simulink model "volo_agcdc_pipelined"  (R2012b)
settings: Solver=ode45  StartTime=0.0  StopTime=1000  RelTol=1e-3
PreLoadFcn:
  | volo_agcdc_init
InitFcn:
  | volo_agcdc_init
StartFcn:
  | volo_agcdc_init
values from neighbouring files (symbols this model uses):
  agc_idleState = 0    [volo_agcdc_init.m]
  agc_numAddrBits = agc_numOutputs + agc_numStateBits    [volo_agcdc_init.m]
  regDCRemoval_AvgLength = 64    [volo_agcdc_init.m]
  regSatDet_NumSamples = 16    [volo_agcdc_init.m]
undefined symbols (not defined in the file or in its folder): gcbh, xlBlockLoadCallback, xlGetNormalizedPeriod
libraries: xbsIndex_r4 x681, xbsEDKLib_r4 x1
(part 2 of 7)

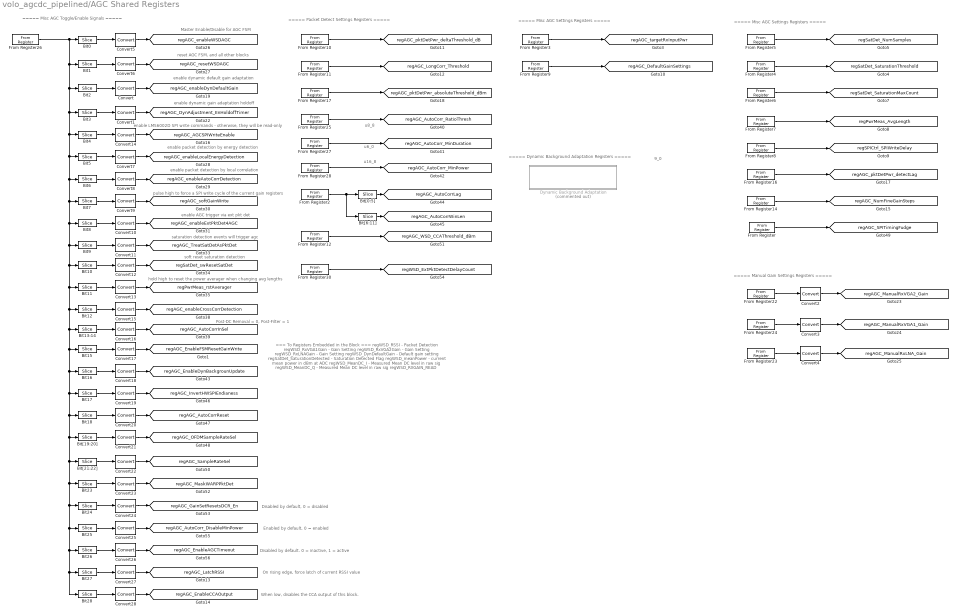
== system volo_agcdc_pipelined/AGC Shared Registers ==
  note: When low, disables the CCA output of this block.
  note: On rising edge, force latch of current RSSI value
  note: Disabled by default, 0 = disabled
  note: Enabled by default, 0 = enabled
  note: Disabled by default. 0 = inactive, 1 = active
  note: u6_0
  note: u16_8
  note: u8_8
  note: 9_0
  note: Post-DC Removal = 0, Post-Filter = 1
  note: ===== Misc AGC Toggle/Enable Signals =====
  note: ===== Dynamic Background Adaptation Registers =====
  note: ===== Misc AGC Settings Registers =====
  note: ===== Misc AGC Settings Registers =====
  note: ===== Packet Detect Settings Registers =====
  note: ===== Manual Gain Settings Registers =====
  note: saturation detection events will trigger agc
  note: enable AGC trigger via ext pkt det
  note: pulse high to force a SPI write cycle of the current gain registers
  note: enable packet detection by local correlation
  note: enable packet detection by energy detection
  note: enable LMS6002D SPI write commands - otherwise, they will be read-only
  note: enable dynamic gain adaptation holdoff
  note: enable dynamic default gain adaptation
  note: reset AGC FSM, and all other blocks
  note: Master Enable/Disable for AGC FSM
  note: === To Registers Embedded in the Block ===
      |
      | regWSD_RSSI - Packet Detection
      | regWSD_RxVGA1Gain - Gain Setting
      | regWSD_RxVGA2Gain - Gain Setting
      | regWSD_RxLNAGain - Gain Setting
      | regWSD_DynDefaultGain - Default gain setting
      | regSatDet_SaturationDetected - Saturation Detected Flag
      | regWSD_meanPower - current mean power in dBm at ADC
      | regWSD_MeanDC_I - Measured Mean DC level in raw sig
      | regWSD_MeanDC_Q - Measured Mean DC level in raw sig
      | regWSD_RXGAIN_READ
  note: soft reset saturation detection
  note: hold high to reset the power averager when changing avg lengths
  Bit0 : xbsIndex_r4/Slice  nbits=1  boolean_output=off  mode=Lower Bit Location + Width  bit1=0  base1=MSB of Input  bit0=0  base0=LSB of Input  dbl_ovrd=off  block_type=slice
  Bit1 : xbsIndex_r4/Slice  nbits=1  boolean_output=off  mode=Lower Bit Location + Width  bit1=0  base1=MSB of Input  bit0=1  base0=LSB of Input  dbl_ovrd=off  block_type=slice
  Bit10 : xbsIndex_r4/Slice  nbits=1  boolean_output=off  mode=Lower Bit Location + Width  bit1=0  base1=MSB of Input  bit0=10  base0=LSB of Input  dbl_ovrd=off  block_type=slice
  Bit11 : xbsIndex_r4/Slice  nbits=1  boolean_output=off  mode=Lower Bit Location + Width  bit1=0  base1=MSB of Input  bit0=11  base0=LSB of Input  dbl_ovrd=off  block_type=slice
  Bit12 : xbsIndex_r4/Slice  nbits=1  boolean_output=off  mode=Lower Bit Location + Width  bit1=0  base1=MSB of Input  bit0=12  base0=LSB of Input  dbl_ovrd=off  block_type=slice
  Bit13:14 : xbsIndex_r4/Slice  nbits=2  boolean_output=off  mode=Lower Bit Location + Width  bit1=0  base1=MSB of Input  bit0=13  base0=LSB of Input  dbl_ovrd=off  block_type=slice
  Bit15 : xbsIndex_r4/Slice  nbits=1  boolean_output=off  mode=Lower Bit Location + Width  bit1=0  base1=MSB of Input  bit0=15  base0=LSB of Input  dbl_ovrd=off  block_type=slice
  Bit16 : xbsIndex_r4/Slice  nbits=1  boolean_output=off  mode=Lower Bit Location + Width  bit1=0  base1=MSB of Input  bit0=16  base0=LSB of Input  dbl_ovrd=off  block_type=slice
  Bit17 : xbsIndex_r4/Slice  nbits=1  boolean_output=off  mode=Lower Bit Location + Width  bit1=0  base1=MSB of Input  bit0=17  base0=LSB of Input  dbl_ovrd=off  block_type=slice
  Bit18 : xbsIndex_r4/Slice  nbits=1  boolean_output=off  mode=Lower Bit Location + Width  bit1=0  base1=MSB of Input  bit0=18  base0=LSB of Input  dbl_ovrd=off  block_type=slice
  Bit2 : xbsIndex_r4/Slice  nbits=1  boolean_output=off  mode=Lower Bit Location + Width  bit1=0  base1=MSB of Input  bit0=2  base0=LSB of Input  dbl_ovrd=off  block_type=slice
  Bit23 : xbsIndex_r4/Slice  nbits=1  boolean_output=off  mode=Lower Bit Location + Width  bit1=0  base1=MSB of Input  bit0=23  base0=LSB of Input  dbl_ovrd=off  block_type=slice
  Bit24 : xbsIndex_r4/Slice  nbits=1  boolean_output=off  mode=Lower Bit Location + Width  bit1=0  base1=MSB of Input  bit0=24  base0=LSB of Input  dbl_ovrd=off  block_type=slice
  Bit25 : xbsIndex_r4/Slice  nbits=1  boolean_output=off  mode=Lower Bit Location + Width  bit1=0  base1=MSB of Input  bit0=25  base0=LSB of Input  dbl_ovrd=off  block_type=slice
  Bit26 : xbsIndex_r4/Slice  nbits=1  boolean_output=off  mode=Lower Bit Location + Width  bit1=0  base1=MSB of Input  bit0=26  base0=LSB of Input  dbl_ovrd=off  block_type=slice
  Bit27 : xbsIndex_r4/Slice  nbits=1  boolean_output=off  mode=Lower Bit Location + Width  bit1=0  base1=MSB of Input  bit0=27  base0=LSB of Input  dbl_ovrd=off  block_type=slice
  Bit28 : xbsIndex_r4/Slice  nbits=1  boolean_output=off  mode=Lower Bit Location + Width  bit1=0  base1=MSB of Input  bit0=28  base0=LSB of Input  dbl_ovrd=off  block_type=slice
  Bit3 : xbsIndex_r4/Slice  nbits=1  boolean_output=off  mode=Lower Bit Location + Width  bit1=0  base1=MSB of Input  bit0=3  base0=LSB of Input  dbl_ovrd=off  block_type=slice
  Bit4 : xbsIndex_r4/Slice  nbits=1  boolean_output=off  mode=Lower Bit Location + Width  bit1=0  base1=MSB of Input  bit0=4  base0=LSB of Input  dbl_ovrd=off  block_type=slice
  Bit5 : xbsIndex_r4/Slice  nbits=1  boolean_output=off  mode=Lower Bit Location + Width  bit1=0  base1=MSB of Input  bit0=5  base0=LSB of Input  dbl_ovrd=off  block_type=slice
  Bit6 : xbsIndex_r4/Slice  nbits=1  boolean_output=off  mode=Lower Bit Location + Width  bit1=0  base1=MSB of Input  bit0=6  base0=LSB of Input  dbl_ovrd=off  block_type=slice
  Bit7 : xbsIndex_r4/Slice  nbits=1  boolean_output=off  mode=Lower Bit Location + Width  bit1=0  base1=MSB of Input  bit0=7  base0=LSB of Input  dbl_ovrd=off  block_type=slice
  Bit8 : xbsIndex_r4/Slice  nbits=1  boolean_output=off  mode=Lower Bit Location + Width  bit1=0  base1=MSB of Input  bit0=8  base0=LSB of Input  dbl_ovrd=off  block_type=slice
  Bit9 : xbsIndex_r4/Slice  nbits=1  boolean_output=off  mode=Lower Bit Location + Width  bit1=0  base1=MSB of Input  bit0=9  base0=LSB of Input  dbl_ovrd=off  block_type=slice
  Bit[0:5] : xbsIndex_r4/Slice  nbits=6  boolean_output=off  mode=Lower Bit Location + Width  bit1=0  base1=MSB of Input  bit0=0  base0=LSB of Input  dbl_ovrd=off  block_type=slice
  Bit[19:20] : xbsIndex_r4/Slice  nbits=2  boolean_output=off  mode=Lower Bit Location + Width  bit1=0  base1=MSB of Input  bit0=19  base0=LSB of Input  dbl_ovrd=off  block_type=slice
  Bit[21:22] : xbsIndex_r4/Slice  nbits=2  boolean_output=off  mode=Lower Bit Location + Width  bit1=0  base1=MSB of Input  bit0=21  base0=LSB of Input  dbl_ovrd=off  block_type=slice
  Bit[6:11] : xbsIndex_r4/Slice  nbits=6  boolean_output=off  mode=Lower Bit Location + Width  bit1=0  base1=MSB of Input  bit0=6  base0=LSB of Input  dbl_ovrd=off  block_type=slice
  Convert{,1,5..15} (13 alike) : xbsIndex_r4/Convert  gui_display_data_type=Boolean  arith_type=Boolean  n_bits=16  bin_pt=14  float_type=Single  exp_bits=8  fraction_bits=24  quantization=Truncate  overflow=Wrap  en=off  latency=0  dbl_ovrd=off  pipeline=off  block_type=convert
  Convert16 : xbsIndex_r4/Convert  gui_display_data_type=Fixed-point  arith_type=Unsigned  n_bits=1  bin_pt=0  float_type=Single  exp_bits=8  fraction_bits=24  quantization=Truncate  overflow=Wrap  en=off  latency=0  dbl_ovrd=off  pipeline=off  block_type=convert
  Convert{17..20,23..28} (10 alike) : xbsIndex_r4/Convert  gui_display_data_type=Boolean  arith_type=Boolean  n_bits=2  bin_pt=0  float_type=Single  exp_bits=8  fraction_bits=24  quantization=Truncate  overflow=Wrap  en=off  latency=0  dbl_ovrd=off  pipeline=off  block_type=convert
  Convert2 : xbsIndex_r4/Convert  gui_display_data_type=Fixed-point  arith_type=Unsigned  n_bits=8  bin_pt=0  float_type=Single  exp_bits=8  fraction_bits=24  quantization=Truncate  overflow=Wrap  en=off  latency=0  dbl_ovrd=off  pipeline=off  block_type=convert
  Convert21 : xbsIndex_r4/Convert  gui_display_data_type=Fixed-point  arith_type=Unsigned  n_bits=2  bin_pt=0  float_type=Single  exp_bits=8  fraction_bits=24  quantization=Truncate  overflow=Wrap  en=off  latency=0  dbl_ovrd=off  pipeline=off  block_type=convert
  Convert22 : xbsIndex_r4/Convert  gui_display_data_type=Fixed-point  arith_type=Unsigned  n_bits=2  bin_pt=0  float_type=Single  exp_bits=8  fraction_bits=24  quantization=Truncate  overflow=Wrap  en=off  latency=0  dbl_ovrd=off  pipeline=off  block_type=convert
  Convert3 : xbsIndex_r4/Convert  gui_display_data_type=Fixed-point  arith_type=Unsigned  n_bits=8  bin_pt=0  float_type=Single  exp_bits=8  fraction_bits=24  quantization=Truncate  overflow=Wrap  en=off  latency=0  dbl_ovrd=off  pipeline=off  block_type=convert
  Convert4 : xbsIndex_r4/Convert  gui_display_data_type=Fixed-point  arith_type=Unsigned  n_bits=8  bin_pt=0  float_type=Single  exp_bits=8  fraction_bits=24  quantization=Truncate  overflow=Wrap  en=off  latency=0  dbl_ovrd=off  pipeline=off  block_type=convert
  Dynamic Background Adaptation : Subsystem  Commented=on
  From Register : xbsIndex_r4/From Register  shared_memory_name='regAGC_SPITIMINGFUDGE'  init=68  period=1  ownership=Locally owned and initialized  gui_display_data_type=Fixed-point  arith_type=Unsigned  n_bits=12  bin_pt=0  preci_type=Single  dbl_ovrd=off  block_type=fromreg
      settings: AttributesFormatString=<< %<shared_memory_name> >>  infoedit="Register block that reads data to a shared memory register.  Delay of one sample period."
  From Register10 : xbsIndex_r4/From Register  shared_memory_name='regAGC_pktDetPwr_deltaThreshold_dBm'  init=regAGC_pktDetPwr_deltaThreshold_dBm  period=1  ownership=Locally owned and initialized  gui_display_data_type=Fixed-point  arith_type="Signed  (2's comp)"  n_bits=9  bin_pt=0  preci_type=Single  dbl_ovrd=off  block_type=fromreg
      settings: AttributesFormatString=<< %<shared_memory_name> >>  infoedit="Register block that reads data to a shared memory register.  Delay of one sample period."
  From Register11 : xbsIndex_r4/From Register  shared_memory_name='regAGC_LongCorr_Threshold'  init=regAGC_LongCorr_Threshold  period=1  ownership=Locally owned and initialized  gui_display_data_type=Fixed-point  arith_type=Unsigned  n_bits=32  bin_pt=0  preci_type=Single  dbl_ovrd=off  block_type=fromreg
      settings: AttributesFormatString=<< %<shared_memory_name> >>  infoedit="Register block that reads data to a shared memory register.  Delay of one sample period."
  From Register12 : xbsIndex_r4/From Register  shared_memory_name='regAGC_WSD_CCAThreshold_dBm'  init=-40  period=1  ownership=Locally owned and initialized  gui_display_data_type=Fixed-point  arith_type=Unsigned  n_bits=10  bin_pt=0  preci_type=Single  dbl_ovrd=off  block_type=fromreg
      settings: AttributesFormatString=<< %<shared_memory_name> >>  infoedit="Register block that reads data to a shared memory register.  Delay of one sample period."
  From Register14 : xbsIndex_r4/From Register  shared_memory_name='regAGC_NumFineGainSteps'  init=regAGC_NumFineGainSteps  period=1  ownership=Locally owned and initialized  gui_display_data_type=Fixed-point  arith_type=Unsigned  n_bits=4  bin_pt=0  preci_type=Single  dbl_ovrd=off  block_type=fromreg
      settings: AttributesFormatString=<< %<shared_memory_name> >>  infoedit="Register block that reads data to a shared memory register.  Delay of one sample period."
  From Register16 : xbsIndex_r4/From Register  shared_memory_name='regAGC_pktDetPwr_detectLag'  init=regAGC_pktDetPwr_detectLag  period=1  ownership=Locally owned and initialized  gui_display_data_type=Fixed-point  arith_type=Unsigned  n_bits=6  bin_pt=0  preci_type=Single  dbl_ovrd=off  block_type=fromreg
      settings: AttributesFormatString=<< %<shared_memory_name> >>  infoedit="Register block that reads data to a shared memory register.  Delay of one sample period."
  From Register17 : xbsIndex_r4/From Register  shared_memory_name='regAGC_pktDetPwr_absoluteThreshold_dBm'  init=regAGC_pktDetPwr_absoluteThreshold_dBm  period=1  ownership=Locally owned and initialized  gui_display_data_type=Fixed-point  arith_type="Signed  (2's comp)"  n_bits=9  bin_pt=0  preci_type=Single  dbl_ovrd=off  block_type=fromreg
      settings: AttributesFormatString=<< %<shared_memory_name> >>  infoedit="Register block that reads data to a shared memory register.  Delay of one sample period."
  From Register2 : xbsIndex_r4/From Register  shared_memory_name='regAGC_AutoCorr_LagTime'  init=16*2^6 + 16  period=2  ownership=Locally owned and initialized  gui_display_data_type=Fixed-point  arith_type=Unsigned  n_bits=12  bin_pt=0  preci_type=Single  dbl_ovrd=off  block_type=fromreg
      settings: AttributesFormatString=<< %<shared_memory_name> >>  infoedit="Register block that reads data to a shared memory register.  Delay of one sample period."
  From Register22 : xbsIndex_r4/From Register  shared_memory_name='regAGC_ManualRxVGA2_Gain'  init=regAGC_ManualRxVGA2_Gain  period=1  ownership=Locally owned and initialized  gui_display_data_type=Fixed-point  arith_type=Unsigned  n_bits=8  bin_pt=0  preci_type=Single  dbl_ovrd=off  block_type=fromreg
      settings: AttributesFormatString=<< %<shared_memory_name> >>  infoedit="Register block that reads data to a shared memory register.  Delay of one sample period."
  From Register23 : xbsIndex_r4/From Register  shared_memory_name='regAGC_ManualRxLNA_Gain'  init=regAGC_ManualRxLNA_Gain  period=1  ownership=Locally owned and initialized  gui_display_data_type=Fixed-point  arith_type=Unsigned  n_bits=8  bin_pt=0  preci_type=Single  dbl_ovrd=off  block_type=fromreg
      settings: AttributesFormatString=<< %<shared_memory_name> >>  infoedit="Register block that reads data to a shared memory register.  Delay of one sample period."
  From Register24 : xbsIndex_r4/From Register  shared_memory_name='regAGC_ManualRxVGA1_Gain'  init=regAGC_ManualRxVGA1_Gain  period=1  ownership=Locally owned and initialized  gui_display_data_type=Fixed-point  arith_type=Unsigned  n_bits=8  bin_pt=0  preci_type=Single  dbl_ovrd=off  block_type=fromreg
      settings: AttributesFormatString=<< %<shared_memory_name> >>  infoedit="Register block that reads data to a shared memory register.  Delay of one sample period."
  From Register25 : xbsIndex_r4/From Register  shared_memory_name='regAGC_AutoCorr_RatioThresh'  init=90  period=1  ownership=Locally owned and initialized  gui_display_data_type=Fixed-point  arith_type=Unsigned  n_bits=8  bin_pt=8  preci_type=Single  dbl_ovrd=off  block_type=fromreg
      settings: AttributesFormatString=<< %<shared_memory_name> >>  infoedit="Register block that reads data to a shared memory register.  Delay of one sample period."
  From Register26 : xbsIndex_r4/From Register  shared_memory_name='regAGC_WSDAGCCtrl'  init=0  period=1  ownership=Locally owned and initialized  gui_display_data_type=Fixed-point  arith_type=Unsigned  n_bits=32  bin_pt=0  preci_type=Single  dbl_ovrd=off  block_type=fromreg
      settings: AttributesFormatString=<< %<shared_memory_name> >>  infoedit="Register block that reads data to a shared memory register.  Delay of one sample period."
  From Register27 : xbsIndex_r4/From Register  shared_memory_name='regAGC_AutoCorr_MinPktDuration'  init=42  period=1  ownership=Locally owned and initialized  gui_display_data_type=Fixed-point  arith_type=Unsigned  n_bits=6  bin_pt=0  preci_type=Single  dbl_ovrd=off  block_type=fromreg
      settings: AttributesFormatString=<< %<shared_memory_name> >>  infoedit="Register block that reads data to a shared memory register.  Delay of one sample period."
  From Register28 : xbsIndex_r4/From Register  shared_memory_name='regAGC_AutoCorr_MinPower'  init=1  period=1  ownership=Locally owned and initialized  gui_display_data_type=Fixed-point  arith_type=Unsigned  n_bits=16  bin_pt=8  preci_type=Single  dbl_ovrd=off  block_type=fromreg
      settings: AttributesFormatString=<< %<shared_memory_name> >>  infoedit="Register block that reads data to a shared memory register.  Delay of one sample period."
  From Register3 : xbsIndex_r4/From Register  shared_memory_name='regAGC_targetRxInputPwr'  init=regAGC_targetRxInputPwr  period=1  ownership=Locally owned and initialized  gui_display_data_type=Fixed-point  arith_type="Signed  (2's comp)"  n_bits=9  bin_pt=0  preci_type=Single  dbl_ovrd=off  block_type=fromreg
      settings: AttributesFormatString=<< %<shared_memory_name> >>  infoedit="Register block that reads data to a shared memory register.  Delay of one sample period."
  From Register30 : xbsIndex_r4/From Register  shared_memory_name='regAGC_ExtPktDet_DelayCount'  init=1  period=1  ownership=Locally owned and initialized  gui_display_data_type=Fixed-point  arith_type=Unsigned  n_bits=32  bin_pt=0  preci_type=Single  dbl_ovrd=off  block_type=fromreg
      settings: AttributesFormatString=<< %<shared_memory_name> >>  infoedit="Register block that reads data to a shared memory register.  Delay of one sample period."
  From Register4 : xbsIndex_r4/From Register  shared_memory_name='regSatDet_SaturationThreshold'  init=regSatDet_SaturationThreshold  period=1  ownership=Locally owned and initialized  gui_display_data_type=Fixed-point  arith_type="Signed  (2's comp)"  n_bits=14  bin_pt=13  preci_type=Single  dbl_ovrd=off  block_type=fromreg
      settings: AttributesFormatString=<< %<shared_memory_name> >>  infoedit="Register block that reads data to a shared memory register.  Delay of one sample period."
  From Register5 : xbsIndex_r4/From Register  shared_memory_name='regSatDet_NumSamples'  init=regSatDet_NumSamples  period=1  ownership=Locally owned and initialized  gui_display_data_type=Fixed-point  arith_type=Unsigned  n_bits=ceil(log(regSatDet_NumSamples)/log(2))+1  bin_pt=0  preci_type=Single  dbl_ovrd=off  block_type=fromreg
      settings: AttributesFormatString=<< %<shared_memory_name> >>  infoedit="Register block that reads data to a shared memory register.  Delay of one sample period."
  From Register6 : xbsIndex_r4/From Register  shared_memory_name='regSatDet_SaturationMaxCount'  init=regSatDet_SaturationMaxCount  period=1  ownership=Locally owned and initialized  gui_display_data_type=Fixed-point  arith_type=Unsigned  n_bits=ceil(log(regSatDet_NumSamples)/log(2)) + 2  bin_pt=0  preci_type=Single  dbl_ovrd=off  block_type=fromreg
      settings: AttributesFormatString=<< %<shared_memory_name> >>  infoedit="Register block that reads data to a shared memory register.  Delay of one sample period."
  From Register7 : xbsIndex_r4/From Register  shared_memory_name='regPwrMeas_AvgLength'  init=regPwrMeas_AvgLength  period=1  ownership=Locally owned and initialized  gui_display_data_type=Fixed-point  arith_type=Unsigned  n_bits=7  bin_pt=0  preci_type=Single  dbl_ovrd=off  block_type=fromreg
      settings: AttributesFormatString=<< %<shared_memory_name> >>  infoedit="Register block that reads data to a shared memory register.  Delay of one sample period."
  From Register8 : xbsIndex_r4/From Register  shared_memory_name='regSPICtrl_SPIWriteDelay'  init=regSPICtrl_SPIWriteDelay  period=1  ownership=Locally owned and initialized  gui_display_data_type=Fixed-point  arith_type=Unsigned  n_bits=8  bin_pt=0  preci_type=Single  dbl_ovrd=off  block_type=fromreg
      settings: AttributesFormatString=<< %<shared_memory_name> >>  infoedit="Register block that reads data to a shared memory register.  Delay of one sample period."
  From Register9 : xbsIndex_r4/From Register  shared_memory_name='regAGC_DefaultGainSettings'  init=regAGC_DefaultGainSettings  period=1  ownership=Locally owned and initialized  gui_display_data_type=Fixed-point  arith_type=Unsigned  n_bits=32  bin_pt=0  preci_type=Single  dbl_ovrd=off  block_type=fromreg
      settings: AttributesFormatString=<< %<shared_memory_name> >>  infoedit="Register block that reads data to a shared memory register.  Delay of one sample period."
  tag scope: regAGC_AGCSPIWriteEnable=global, regAGC_AutoCorrInSel=global, regAGC_AutoCorrLag=global, regAGC_AutoCorrReset=global, regAGC_AutoCorrWinLen=global, regAGC_AutoCorr_DisableMinPower=global, regAGC_AutoCorr_MinDuration=global, regAGC_AutoCorr_MinPower=global, regAGC_AutoCorr_RatioThresh=global, regAGC_DefaultGainSettings=global, regAGC_DynAdjustment_EnHoldoffTimer=global, regAGC_EnableAGCTimeout=global, regAGC_EnableCCAOutput=global, regAGC_EnableDynBackgrounUpdate=global, regAGC_EnableFSMResetGainWrite=global, regAGC_GainSetResetsDCR_En=global, regAGC_InvertHWSPIEndianess=global, regAGC_LatchRSSI=global, regAGC_LongCorr_Threshold=global, regAGC_ManualRxLNA_Gain=global, regAGC_ManualRxVGA1_Gain=global, regAGC_ManualRxVGA2_Gain=global, regAGC_MaskWARPPktDet=global, regAGC_NumFineGainSteps=global, regAGC_OFDMSampleRateSel=global, regAGC_SPITimingFudge=global, regAGC_SampleRateSel=global, regAGC_TreatSatDetAsPktDet=global, regAGC_WSD_CCAThreshold_dBm=global, regAGC_enableAutoCorrDetection=global, regAGC_enableCrossCorrDetection=global, regAGC_enableDynDefaultGain=global, regAGC_enableExtPktDet4AGC=global, regAGC_enableLocalEnergyDetection=global, regAGC_enableWSDAGC=global, regAGC_pktDetPwr_absoluteThreshold_dBm=global, regAGC_pktDetPwr_deltaThreshold_dB=global, regAGC_pktDetPwr_detectLag=global, regAGC_resetWSDAGC=global, regAGC_softGainWrite=global, regAGC_targetRxInputPwr=global, regPwrMeas_AvgLength=global, regPwrMeas_rstAverager=global, regSPICtrl_SPIWriteDelay=global, regSatDet_NumSamples=global, regSatDet_SaturationMaxCount=global, regSatDet_SaturationThreshold=global, regSatDet_swResetSatDet=global, regWSD_ExtPktDetectDelayCount=global
  wires:
  From Register3/1 -> [regAGC_targetRxInputPwr]
  From Register4/1 -> [regSatDet_SaturationThreshold]
  From Register5/1 -> [regSatDet_NumSamples]
  From Register6/1 -> [regSatDet_SaturationMaxCount]
  From Register7/1 -> [regPwrMeas_AvgLength]
  From Register8/1 -> [regSPICtrl_SPIWriteDelay]
  From Register9/1 -> [regAGC_DefaultGainSettings]
  From Register10/1 -> [regAGC_pktDetPwr_deltaThreshold_dB]
  From Register11/1 -> [regAGC_LongCorr_Threshold]
  From Register14/1 -> [regAGC_NumFineGainSteps]
  From Register17/1 -> [regAGC_pktDetPwr_absoluteThreshold_dBm]
  From Register16/1 -> [regAGC_pktDetPwr_detectLag]
  From Register22/1 -> Convert2/1
  From Register24/1 -> Convert3/1
  Convert3/1 -> [regAGC_ManualRxVGA1_Gain]
  Convert2/1 -> [regAGC_ManualRxVGA2_Gain]
  From Register23/1 -> Convert4/1
  Convert4/1 -> [regAGC_ManualRxLNA_Gain]
  Bit1/1 -> Convert6/1
  Convert5/1 -> [regAGC_enableWSDAGC]
  Convert6/1 -> [regAGC_resetWSDAGC]
  Bit0/1 -> Convert5/1
  Convert/1 -> [regAGC_enableDynDefaultGain]
  Bit2/1 -> Convert/1
  Convert1/1 -> [regAGC_DynAdjustment_EnHoldoffTimer]
  Bit3/1 -> Convert1/1
  Bit4/1 -> Convert14/1
  Convert7/1 -> [regAGC_enableLocalEnergyDetection]
  Bit5/1 -> Convert7/1
  Convert8/1 -> [regAGC_enableAutoCorrDetection]
  Bit6/1 -> Convert8/1
  Convert9/1 -> [regAGC_softGainWrite]
  Bit7/1 -> Convert9/1
  Bit8/1 -> Convert10/1
  Convert10/1 -> [regAGC_enableExtPktDet4AGC]
  Bit9/1 -> Convert11/1
  Convert11/1 -> [regAGC_TreatSatDetAsPktDet]
  Bit10/1 -> Convert12/1
  Convert12/1 -> [regSatDet_swResetSatDet]
  Bit11/1 -> Convert13/1
  Convert13/1 -> [regPwrMeas_rstAverager]
  Convert14/1 -> [regAGC_AGCSPIWriteEnable]
  Bit12/1 -> Convert15/1
  Convert15/1 -> [regAGC_enableCrossCorrDetection]
  Bit13:14/1 -> Convert16/1
  Convert16/1 -> [regAGC_AutoCorrInSel]
  From Register25/1 -> [regAGC_AutoCorr_RatioThresh]
  From Register27/1 -> [regAGC_AutoCorr_MinDuration]
  From Register28/1 -> [regAGC_AutoCorr_MinPower]
  Bit15/1 -> Convert17/1
  Convert17/1 -> [regAGC_EnableFSMResetGainWrite]
  Bit16/1 -> Convert18/1
  Convert18/1 -> [regAGC_EnableDynBackgrounUpdate]
  From Register2/1 -> Bit[6:11]/1, Bit[0:5]/1
  Bit[0:5]/1 -> [regAGC_AutoCorrLag]
  Bit[6:11]/1 -> [regAGC_AutoCorrWinLen]
  Bit17/1 -> Convert19/1
  Convert19/1 -> [regAGC_InvertHWSPIEndianess]
  Bit18/1 -> Convert20/1
  Convert20/1 -> [regAGC_AutoCorrReset]
  Bit[19:20]/1 -> Convert21/1
  Convert21/1 -> [regAGC_OFDMSampleRateSel]
  From Register/1 -> [regAGC_SPITimingFudge]
  Bit[21:22]/1 -> Convert22/1
  Convert22/1 -> [regAGC_SampleRateSel]
  Bit23/1 -> Convert23/1
  Convert23/1 -> [regAGC_MaskWARPPktDet]
  From Register26/1 -> Bit0/1, Bit1/1, Bit17/1, Bit28/1, Bit27/1, Bit26/1, Bit25/1, Bit24/1, Bit23/1, Bit[21:22]/1, Bit[19:20]/1, Bit18/1, Bit16/1, Bit15/1, Bit13:14/1, Bit12/1, Bit11/1, Bit10/1, Bit9/1, Bit8/1, Bit7/1, Bit6/1, Bit5/1, Bit4/1, Bit3/1, Bit2/1
  Bit24/1 -> Convert24/1
  Convert24/1 -> [regAGC_GainSetResetsDCR_En]
  Bit25/1 -> Convert25/1
  Convert25/1 -> [regAGC_AutoCorr_DisableMinPower]
  Bit26/1 -> Convert26/1
  Convert26/1 -> [regAGC_EnableAGCTimeout]
  Bit27/1 -> Convert27/1
  Convert27/1 -> [regAGC_LatchRSSI]
  From Register30/1 -> [regWSD_ExtPktDetectDelayCount]
  Bit28/1 -> Convert28/1
  Convert28/1 -> [regAGC_EnableCCAOutput]
  From Register12/1 -> [regAGC_WSD_CCAThreshold_dBm]

== system volo_agcdc_pipelined/AGC_FSM ==
  note: GetGain_Go is buggy when AGCDone
  note: When AGC_Done is high,
      | freeze state.
  note: Reset line for the Avg. Power block
  note: Pulse to increment the counter for the number
      | of times fine gain has been set.
  note: Reset line for the Saturation Detector
  note: Pulse to trigger a round of gain setting
  note: Finite state machine defined by the state/output transition tables
      | agc_next_state_ROM and agc_output_ROM. Inputs and outputs
      | are a standard Mealy FSM, with the exception that the EnableAGC
      | line is implemented in such a way that overrides the entire state
      | machine. This was done to preserve ROM (otherwise, it's always
      | 2x ROM to add an additional input reset bit). It also ensures that
      | regardless of the correctness of the FSM state/output transition
      | tables, the FSM always starts and resets to a known state.
      |
      | This FSM controls the AGC logic by triggering/resetting saturation
      | detection, power measurement, and gain setting events, and then
      | waiting for those blocks to signal complete before taking action.
      |
      | In hindsight, the ease of debugging and modifiability of this state
      | machine is much better if one increases the number of states. In
      | that case, the state machine is also very sparse. I'm sure there is
      | a much better way to build this, but we're already pot-committed
      | and it takes a very long time to test, debug and tweak.
      | me@ryaneguerra.com
      | May 5, 2013
  EnableAGC : Inport
  SatDet_Good : Inport  Port=2
  SatDet : Inport  Port=3
  SetGainDone : Inport  Port=4
  PwrMeas_Good : Inport  Port=5
  AGC_Done : Inport  Port=6
  Bit0 : xbsIndex_r4/Slice  nbits=1  boolean_output=on  mode=Upper Bit Location + Width  bit1=0  base1=LSB of Input  bit0=0  base0=LSB of Input  dbl_ovrd=off  block_type=slice
  Bit1 : xbsIndex_r4/Slice  nbits=1  boolean_output=on  mode=Upper Bit Location + Width  bit1=1  base1=LSB of Input  bit0=0  base0=LSB of Input  dbl_ovrd=off  block_type=slice
  Bit2 : xbsIndex_r4/Slice  nbits=1  boolean_output=on  mode=Upper Bit Location + Width  bit1=2  base1=LSB of Input  bit0=0  base0=LSB of Input  dbl_ovrd=off  block_type=slice
  Bit3 : xbsIndex_r4/Slice  nbits=1  boolean_output=on  mode=Upper Bit Location + Width  bit1=3  base1=LSB of Input  bit0=0  base0=LSB of Input  dbl_ovrd=off  block_type=slice
  Concat : xbsIndex_r4/Concat  num_inputs=2  dbl_ovrd=off  block_type=concat
      settings: block_version=VER_STRING_GOES_HERE
  Concat1 : xbsIndex_r4/Concat  num_inputs=4  dbl_ovrd=off  block_type=concat
      settings: block_version=VER_STRING_GOES_HERE
  Idle_State : xbsIndex_r4/Constant  const=agc_idleState  gui_display_data_type=Fixed-point  arith_type=Unsigned  n_bits=agc_numStateBits  bin_pt=0  preci_type=Single  exp_width=8  frac_width=24  explicit_period=on  period=1  equ=P=C  opselect=C  inp2=PCIN>>17  opr=+  inp1=P  carry=CIN  dbl_ovrd=off  block_type=constant
  Inverter2 : xbsIndex_r4/Inverter  en=off  latency=0  dbl_ovrd=off  block_type=inv
  Logical1 : xbsIndex_r4/Logical  logical_function=AND  inputs=2  en=off  latency=0  precision=Full  arith_type=Unsigned  n_bits=16  bin_pt=0  align_bp=on  dbl_ovrd=off  block_type=logical
  Mux : xbsIndex_r4/Mux  inputs=2  en=off  latency=0  precision=User Defined  arith_type=Unsigned  n_bits=agc_numStateBits  bin_pt=0  quantization=Truncate  overflow=Saturate  dbl_ovrd=off  block_type=mux
  Mux1 : xbsIndex_r4/Mux  inputs=2  en=off  latency=0  precision=User Defined  arith_type=Unsigned  n_bits=agc_numStateBits  bin_pt=0  quantization=Truncate  overflow=Saturate  dbl_ovrd=off  block_type=mux
  Next_State_ROM : xbsIndex_r4/ROM  depth=2^agc_numAddrBits  initVector=agc_next_state_ROM  distributed_mem=Block RAM  rst=off  init_reg=0  en=off  latency=1  gui_display_data_type=Fixed-point  arith_type=Unsigned  n_bits=agc_numStateBits  bin_pt=0  preci_type=Single  exp_width=8  frac_width=24  dbl_ovrd=off  optimize=Area  use_rpm=on  block_type=sprom
  Output_ROM : xbsIndex_r4/ROM  depth=2^agc_numAddrBits  initVector=agc_output_ROM  distributed_mem=Block RAM  rst=off  init_reg=0  en=off  latency=1  gui_display_data_type=Fixed-point  arith_type=Unsigned  n_bits=agc_numOutputs  bin_pt=0  preci_type=Single  exp_width=8  frac_width=24  dbl_ovrd=off  optimize=Area  use_rpm=on  block_type=sprom
  Register : xbsIndex_r4/Register  init=0  rst=off  en=off  dbl_ovrd=off  block_type=register
  SetGain_Go : Outport
  SatDet_Rst : Outport  Port=2
  PwrSet_Inc : Outport  Port=3
  PwrMeas_Rst : Outport  Port=4
  CurrentState : Outport  Port=5
  tag scope: cs_agc_current_state=global, cs_pwrset_inc=global, cs_setgain_go=global
  wires:
  Concat/1 -> Output_ROM/1, Next_State_ROM/1
  SatDet_Good/1 -> Concat1/1
  SatDet/1 -> Concat1/2
  SetGainDone/1 -> Concat1/3
  PwrMeas_Good/1 -> Concat1/4
  Concat1/1 -> Concat/2
  EnableAGC/1 -> Mux/1
  Next_State_ROM/1 -> Mux/3  "Next_State"
  Mux/1 -> Mux1/2
  Idle_State/1 -> Mux/2
  Output_ROM/1 -> Bit2/1, Bit0/1, Bit1/1, Bit3/1  "Output_Signals"
  Bit3/1 -> Logical1/2  "SetGain_Go"
  Bit2/1 -> SatDet_Rst/1
  Bit1/1 -> [cs_pwrset_inc], PwrSet_Inc/1
  Bit0/1 -> PwrMeas_Rst/1
  Mux1/1 -> [cs_agc_current_state], CurrentState/1, Register/1, Concat/1
  AGC_Done/1 -> Inverter2/1, Mux1/1
  Register/1 -> Mux1/3
  Inverter2/1 -> Logical1/1  "AGC Not done"
  Logical1/1 -> [cs_setgain_go], SetGain_Go/1

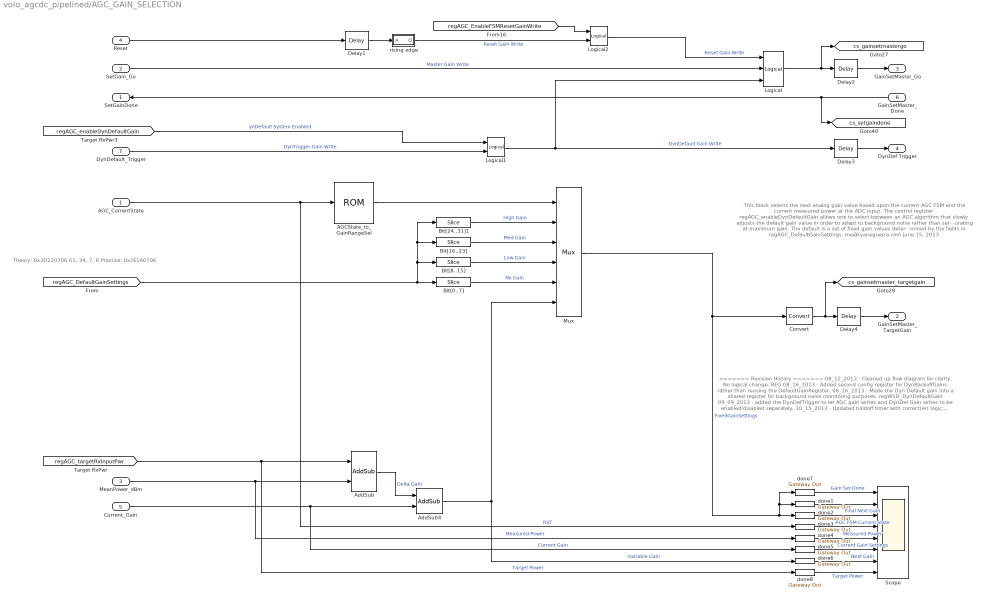
== system volo_agcdc_pipelined/AGC_GAIN_SELECTION ==
  note: Theory: 0x3D220706
      | 61, 34, 7, 6
      | Practice: 0x2E1A0706
  note: ======= Revision History =======
      | 08_12_2013 - Cleaned up flow diagram for clarity. No logical change. REG
      | 08_16_2013 - Added second config register for DynBackoffGains rather than
      | reusing the DefaultGainRegister.
      | 08_16_2013 - Made the Dyn Default gain into a shared register for background noise
      | monitoring purposes. regWSD_DynDefaultGain
      | 09_09_2013 - added the DynDefTrigger to let AGC gain writes and DynDef Gain writes to
      | be enabled/disabled separately.
      | 10_15_2013 - Updated holdoff timer with correct(er) logic; added bounds checking REG
      | 10_23_2013 - Added EnableFSMResetGainWrite to provide software control over whether
      | or not a reset of the FSM (read: when PktDet goes low due to finished or missed packet)
      | writes current gain settings (meant to reset to default gain after AGC). Also updated signal
      | path for DynTrigger Gain Write signal since it wasn't properly masked.
      | 10_23_2013 - Fixed bounds checking--DOH! REG
  note: This block selects the next analog gain value based
      | upon the current AGC FSM and the current measured power
      | at the ADC input. The control register regAGC_enableDynDefaultGain
      | allows one to select between an AGC algorithm that slowly adjusts the
      | default gain value in order to adapt to background noise rather than sat-
      | -urating at maximum gain. The default is a set of fixed gain values deter-
      | -mined by the fields in regAGC_DefaultGainSettings.
      | me@ryaneguerra.com
      | June 15, 2013
  AGC_CurrentState : Inport
  SetGain_Go : Inport  Port=2
  MeanPower_dBm : Inport  Port=3
  Reset : Inport  Port=4
  Current_Gain : Inport  Port=5
  GainSetMaster_Done : Inport  Port=6
  DynDefault_Trigger : Inport  Port=7
  AGCState_to_GainRangeSel : xbsIndex_r4/ROM  depth=8  initVector=[0, 1, 0, 2, 0, 3, 0, 4]  distributed_mem=Block RAM  rst=off  init_reg=0  en=off  latency=1  gui_display_data_type=Fixed-point  arith_type=Unsigned  n_bits=3  bin_pt=0  preci_type=Single  exp_width=8  frac_width=24  dbl_ovrd=off  optimize=Area  use_rpm=on  block_type=sprom
  AddSub : xbsIndex_r4/AddSub  mode=Subtraction  use_carryin=off  use_carryout=off  en=off  latency=0  precision=User Defined  arith_type="Signed  (2's comp)"  n_bits=9  bin_pt=0  quantization=Truncate  overflow=Saturate  dbl_ovrd=off  use_behavioral_HDL=off  hw_selection=Fabric  pipelined=off  block_type=addsub
  AddSub4 : xbsIndex_r4/AddSub  mode=Addition  use_carryin=off  use_carryout=off  en=off  latency=0  precision=User Defined  arith_type="Signed  (2's comp)"  n_bits=9  bin_pt=0  quantization=Truncate  overflow=Saturate  dbl_ovrd=off  use_behavioral_HDL=off  hw_selection=Fabric  pipelined=off  block_type=addsub
  Bit[0..7] : xbsIndex_r4/Slice  nbits=8  boolean_output=off  mode=Lower Bit Location + Width  bit1=0  base1=MSB of Input  bit0=0  base0=LSB of Input  dbl_ovrd=off  block_type=slice
  Bit[16..23] : xbsIndex_r4/Slice  nbits=8  boolean_output=off  mode=Lower Bit Location + Width  bit1=0  base1=MSB of Input  bit0=16  base0=LSB of Input  dbl_ovrd=off  block_type=slice
  Bit[24..31]1 : xbsIndex_r4/Slice  nbits=8  boolean_output=off  mode=Lower Bit Location + Width  bit1=0  base1=MSB of Input  bit0=24  base0=LSB of Input  dbl_ovrd=off  block_type=slice
  Bit[8..15] : xbsIndex_r4/Slice  nbits=8  boolean_output=off  mode=Lower Bit Location + Width  bit1=0  base1=MSB of Input  bit0=8  base0=LSB of Input  dbl_ovrd=off  block_type=slice
  Convert : xbsIndex_r4/Convert  gui_display_data_type=Fixed-point  arith_type=Unsigned  n_bits=6  bin_pt=0  float_type=Single  exp_bits=8  fraction_bits=24  quantization=Truncate  overflow=Saturate  en=off  latency=0  dbl_ovrd=off  pipeline=off  block_type=convert
  Delay1 : xbsIndex_r4/Delay  rst=off  infoeditControl=Selection of Reset will increase slice count due to use of real FFs and instead of SRLs  en=off  latency=3  dbl_ovrd=off  reg_retiming=off  block_type=delay
  Delay2 : xbsIndex_r4/Delay  rst=off  infoeditControl=Selection of Reset will increase slice count due to use of real FFs and instead of SRLs  en=off  latency=1  dbl_ovrd=off  reg_retiming=off  block_type=delay
  Delay3 : xbsIndex_r4/Delay  rst=off  infoeditControl=Selection of Reset will increase slice count due to use of real FFs and instead of SRLs  en=off  latency=1  dbl_ovrd=off  reg_retiming=off  block_type=delay
  Delay4 : xbsIndex_r4/Delay  rst=off  infoeditControl=Selection of Reset will increase slice count due to use of real FFs and instead of SRLs  en=off  latency=1  dbl_ovrd=off  reg_retiming=off  block_type=delay
  Logical : xbsIndex_r4/Logical  logical_function=OR  inputs=3  en=off  latency=0  precision=Full  arith_type=Unsigned  n_bits=16  bin_pt=0  align_bp=on  dbl_ovrd=off  block_type=logical
  Logical1 : xbsIndex_r4/Logical  logical_function=AND  inputs=2  en=off  latency=0  precision=Full  arith_type=Unsigned  n_bits=16  bin_pt=0  align_bp=on  dbl_ovrd=off  block_type=logical
  Logical2 : xbsIndex_r4/Logical  logical_function=AND  inputs=2  en=off  latency=0  precision=Full  arith_type=Unsigned  n_bits=16  bin_pt=0  align_bp=on  dbl_ovrd=off  block_type=logical
  Mux : xbsIndex_r4/Mux  inputs=5  en=off  latency=0  precision=Full  arith_type=Unsigned  n_bits=16  bin_pt=14  quantization=Truncate  overflow=Wrap  dbl_ovrd=off  block_type=mux
  Scope : Scope  NumInputPorts=8
      settings: ShowLegends=on  YMin=-5~-5~-5~-5~-5~-5~-5~-5  YMax=5~5~5~5~5~5~5~5  SaveName=ScopeData3
  done{1..8} (8 alike) : xbsIndex_r4/Gateway Out  inherit_from_input=off  hdl_port=off  timing_constraint=None  locs_specified=off  LOCs={}  UseAsDAC=off  DACChannel='1'  block_type=gatewayout
      settings: infoedit="Gateway out block.  Converts Xilinx fixed point inputs into ouputs of type Simulink integer, double, or fixed point.<P><P>Hardware notes:  In hardware these blocks become top level output ports or are discarded, depending on how they are configured."  xl_area=[0 0 0 0 1 0 0]  block_version=VER_STRING_GOES_HERE
  rising edge : Subsystem
  SetGainDone : Outport
  GainSetMaster_TargetGain : Outport  Port=2
  GainSetMaster_Go : Outport  Port=3
  DynDef Trigger : Outport  Port=4
  tag scope: cs_gainsetmaster_targetgain=global, cs_gainsetmastergo=global, cs_setgaindone=global
  wires:
  done7/1 -> Scope/1  "Gain Set Done"
  done1/1 -> Scope/2
  done2/1 -> Scope/3  "Final Next Gain"
  done3/1 -> Scope/4  "AGC FSM Current State"
  done4/1 -> Scope/5  "Measured Power"
  Bit[8..15]/1 -> Mux/4  "Low Gain"
  Current_Gain/1 -> done5/1, AddSub4/2  "Current Gain"
  [regAGC_targetRxInputPwr] -> AddSub/1, done8/1  "Target Power"
  MeanPower_dBm/1 -> done4/1, AddSub/2  "Measured Power"
  AddSub4/1 -> Mux/6, done6/1  "Variable Gain"
  Bit[0..7]/1 -> Mux/5  "No Gain"
  AGCState_to_GainRangeSel/1 -> Mux/1
  AGC_CurrentState/1 -> done3/1, AGCState_to_GainRangeSel/1  "RST"
  AddSub/1 -> AddSub4/1  "Delta Gain"
  done5/1 -> Scope/6  "Current Gain Settings"
  done6/1 -> Scope/7  "Next Gain"
  done8/1 -> Scope/8  "Target Power"
  [regAGC_DefaultGainSettings] -> Bit[0..7]/1, Bit[8..15]/1, Bit[16..23]/1, Bit[24..31]1/1
  Reset/1 -> Delay1/1
  SetGain_Go/1 -> Logical/2  "Master Gain Write"
  rising edge/1(Q) -> Logical2/2  "Reset Gain Write"
  Convert/1 -> [cs_gainsetmaster_targetgain], Delay4/1
  Logical/1 -> [cs_gainsetmastergo], Delay2/1
  Delay1/1 -> rising edge/1(A)
  DynDefault_Trigger/1 -> Logical1/2  "DynTrigger Gain Write"
  Bit[24..31]1/1 -> Mux/2  "High Gain"
  Bit[16..23]/1 -> Mux/3  "Med Gain"
  Mux/1 -> Convert/1, done2/1, done7/1, done1/1  "FixedGainSettings"
  [regAGC_enableDynDefaultGain] -> Logical1/1  "ynDefault System Enabled"
  Logical1/1 -> Logical/3, Delay3/1  "DynDefault Gain Write"
  Logical2/1 -> Logical/1  "Reset Gain Write"
  [regAGC_EnableFSMResetGainWrite] -> Logical2/1
  Delay2/1 -> GainSetMaster_Go/1
  GainSetMaster_Done/1 -> [cs_setgaindone], SetGainDone/1
  Delay4/1 -> GainSetMaster_TargetGain/1
  Delay3/1 -> DynDef Trigger/1

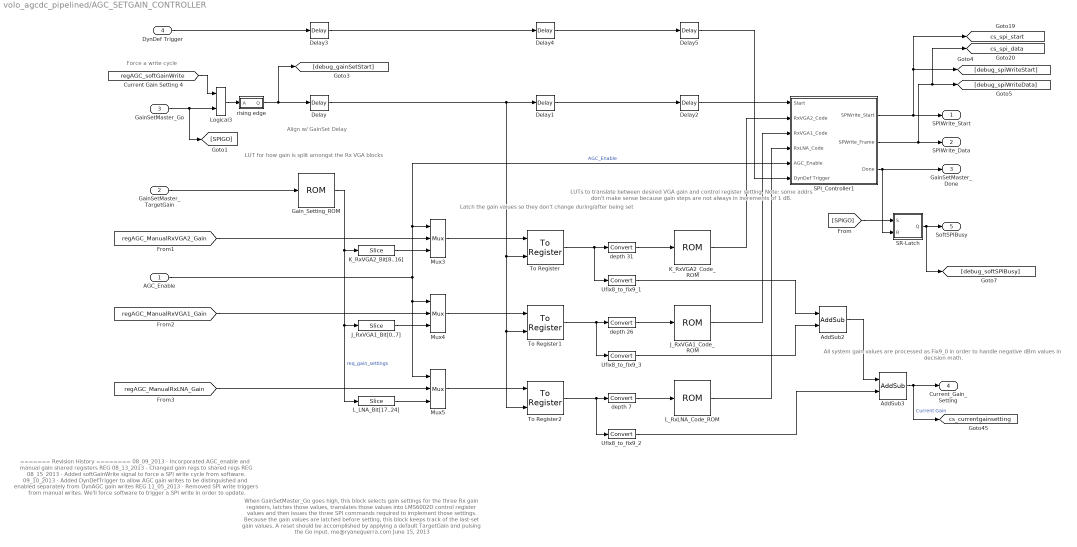
== system volo_agcdc_pipelined/AGC_SETGAIN_CONTROLLER ==
  note: Align w/ GainSet Delay
  note: Force a write cycle
  note: ======= Revision History ========
      | 08_09_2013 - Incorporated AGC_enable and
      | manual gain shared registers REG
      | 08_13_2013 - Changed gain regs to shared regs REG
      | 08_15_2013 - Added softGainWrite signal to force a SPI write cycle
      | from software.
      | 09_10_2013 - Added DynDefTrigger to allow AGC gain writes to be
      | distinguished and enabled separately from DynAGC gain writes REG
      | 11_05_2013 - Removed SPI write triggers from manual writes. We'll
      | force software to trigger a SPI write in order to update.
  note: When GainSetMaster_Go goes high, this block selects gain settings for the three Rx gain
      | registers, latches those values, translates those values into LMS6002D control register values
      | and then issues the three SPI commands required to implement those settings. Because the
      | gain values are latched before setting, this block keeps track of the last-set gain values. A reset
      | should be accomplished by applying a default TargetGain and pulsing the Go input.
      | me@ryaneguerra.com
      | June 15, 2013
  note: Latch the gain values
      | so they don't change
      | during/after being set
  note: LUTs to translate between
      | desired VGA gain and control
      | register setting. Note: some
      | addrs don't make sense because
      | gain steps are not always in
      | increments of 1 dB.
  note: LUT for how gain
      | is split amongst the
      | Rx VGA blocks
  note: All system gain values are processed as Fix9_0
      | in order to handle negative dBm values in decision
      | math.
  AGC_Enable : Inport
  GainSetMaster_TargetGain : Inport  Port=2
  GainSetMaster_Go : Inport  Port=3
  DynDef Trigger : Inport  Port=4
  AddSub2 : xbsIndex_r4/AddSub  mode=Addition  use_carryin=off  use_carryout=off  en=off  latency=0  precision=User Defined  arith_type="Signed  (2's comp)"  n_bits=9  bin_pt=0  quantization=Truncate  overflow=Saturate  dbl_ovrd=off  use_behavioral_HDL=off  hw_selection=Fabric  pipelined=off  block_type=addsub
  AddSub3 : xbsIndex_r4/AddSub  mode=Addition  use_carryin=off  use_carryout=off  en=off  latency=0  precision=User Defined  arith_type="Signed  (2's comp)"  n_bits=9  bin_pt=0  quantization=Truncate  overflow=Saturate  dbl_ovrd=off  use_behavioral_HDL=off  hw_selection=Fabric  pipelined=off  block_type=addsub
  Delay{,1..5} (6 alike) : xbsIndex_r4/Delay  rst=off  infoeditControl=Selection of Reset will increase slice count due to use of real FFs and instead of SRLs  en=off  latency=1  dbl_ovrd=off  reg_retiming=off  block_type=delay
  Gain_Setting_ROM : xbsIndex_r4/ROM  depth=64  initVector=GAIN_ROM  distributed_mem=Block RAM  rst=off  init_reg=0  en=off  latency=1  gui_display_data_type=Fixed-point  arith_type=Unsigned  n_bits=32  bin_pt=0  preci_type=Single  exp_width=8  frac_width=24  dbl_ovrd=off  optimize=Speed  use_rpm=on  block_type=sprom
  J_RxVGA1_Bit[0..7] : xbsIndex_r4/Slice  nbits=8  boolean_output=off  mode=Lower Bit Location + Width  bit1=0  base1=MSB of Input  bit0=0  base0=LSB of Input  dbl_ovrd=off  block_type=slice
  J_RxVGA1_Code_ROM : xbsIndex_r4/ROM  depth=26  initVector=J_RxVGA1_CODE_ROM  distributed_mem=Block RAM  rst=off  init_reg=0  en=off  latency=1  gui_display_data_type=Fixed-point  arith_type=Unsigned  n_bits=8  bin_pt=0  preci_type=Single  exp_width=8  frac_width=24  dbl_ovrd=off  optimize=Speed  use_rpm=on  block_type=sprom
  K_RxVGA2_Bit[8..16] : xbsIndex_r4/Slice  nbits=8  boolean_output=off  mode=Lower Bit Location + Width  bit1=0  base1=MSB of Input  bit0=8  base0=LSB of Input  dbl_ovrd=off  block_type=slice
  K_RxVGA2_Code_ROM : xbsIndex_r4/ROM  depth=31  initVector=K_RxVGA2_CODE_ROM  distributed_mem=Block RAM  rst=off  init_reg=0  en=off  latency=1  gui_display_data_type=Fixed-point  arith_type=Unsigned  n_bits=8  bin_pt=0  preci_type=Single  exp_width=8  frac_width=24  dbl_ovrd=off  optimize=Speed  use_rpm=on  block_type=sprom
  L_LNA_Bit[17..24] : xbsIndex_r4/Slice  nbits=8  boolean_output=off  mode=Lower Bit Location + Width  bit1=0  base1=MSB of Input  bit0=16  base0=LSB of Input  dbl_ovrd=off  block_type=slice
  L_RxLNA_Code_ROM : xbsIndex_r4/ROM  depth=7  initVector=L_RxLNA_CODE_ROM  distributed_mem=Block RAM  rst=off  init_reg=0  en=off  latency=1  gui_display_data_type=Fixed-point  arith_type=Unsigned  n_bits=8  bin_pt=0  preci_type=Single  exp_width=8  frac_width=24  dbl_ovrd=off  optimize=Speed  use_rpm=on  block_type=sprom
  Logical3 : xbsIndex_r4/Logical  logical_function=OR  inputs=2  en=off  latency=0  precision=Full  arith_type=Unsigned  n_bits=16  bin_pt=0  align_bp=on  dbl_ovrd=off  block_type=logical
  Mux3 : xbsIndex_r4/Mux  inputs=2  en=off  latency=0  precision=Full  arith_type=Unsigned  n_bits=16  bin_pt=14  quantization=Truncate  overflow=Wrap  dbl_ovrd=off  block_type=mux
  Mux4 : xbsIndex_r4/Mux  inputs=2  en=off  latency=0  precision=Full  arith_type=Unsigned  n_bits=16  bin_pt=14  quantization=Truncate  overflow=Wrap  dbl_ovrd=off  block_type=mux
  Mux5 : xbsIndex_r4/Mux  inputs=2  en=off  latency=0  precision=Full  arith_type=Unsigned  n_bits=16  bin_pt=14  quantization=Truncate  overflow=Wrap  dbl_ovrd=off  block_type=mux
  SPI_Controller1 : Subsystem
  SR-Latch : Subsystem
  To Register : xbsIndex_r4/To Register  shared_memory_name='regWSD_RxVGA2Gain'  init=0  ownership=Locally owned and initialized  explicit_data_type=on  gui_display_data_type=Fixed-point  arith_type=Unsigned  n_bits=8  bin_pt=0  preci_type=Single  dbl_ovrd=off  block_type=toreg
      settings: AttributesFormatString=<< %<shared_memory_name> >>  infoedit="Register block that writes data to a shared memory register.  Delay of one sample period."
  To Register1 : xbsIndex_r4/To Register  shared_memory_name='regWSD_RxVGA1Gain'  init=0  ownership=Locally owned and initialized  explicit_data_type=on  gui_display_data_type=Fixed-point  arith_type=Unsigned  n_bits=8  bin_pt=0  preci_type=Single  dbl_ovrd=off  block_type=toreg
      settings: AttributesFormatString=<< %<shared_memory_name> >>  infoedit="Register block that writes data to a shared memory register.  Delay of one sample period."
  To Register2 : xbsIndex_r4/To Register  shared_memory_name='regWSD_RxLNAGain'  init=6  ownership=Locally owned and initialized  explicit_data_type=on  gui_display_data_type=Fixed-point  arith_type=Unsigned  n_bits=8  bin_pt=0  preci_type=Single  dbl_ovrd=off  block_type=toreg
      settings: AttributesFormatString=<< %<shared_memory_name> >>  infoedit="Register block that writes data to a shared memory register.  Delay of one sample period."
  Ufix8_to_fix9_1 : xbsIndex_r4/Convert  gui_display_data_type=Fixed-point  arith_type="Signed  (2's comp)"  n_bits=9  bin_pt=0  float_type=Single  exp_bits=8  fraction_bits=24  quantization=Truncate  overflow=Saturate  en=off  latency=0  dbl_ovrd=off  pipeline=off  block_type=convert
  Ufix8_to_fix9_2 : xbsIndex_r4/Convert  gui_display_data_type=Fixed-point  arith_type="Signed  (2's comp)"  n_bits=9  bin_pt=0  float_type=Single  exp_bits=8  fraction_bits=24  quantization=Truncate  overflow=Saturate  en=off  latency=0  dbl_ovrd=off  pipeline=off  block_type=convert
  Ufix8_to_fix9_3 : xbsIndex_r4/Convert  gui_display_data_type=Fixed-point  arith_type="Signed  (2's comp)"  n_bits=9  bin_pt=0  float_type=Single  exp_bits=8  fraction_bits=24  quantization=Truncate  overflow=Saturate  en=off  latency=0  dbl_ovrd=off  pipeline=off  block_type=convert
  depth 26 : xbsIndex_r4/Convert  gui_display_data_type=Fixed-point  arith_type=Unsigned  n_bits=5  bin_pt=0  float_type=Single  exp_bits=8  fraction_bits=24  quantization=Truncate  overflow=Saturate  en=off  latency=0  dbl_ovrd=off  pipeline=off  block_type=convert
  depth 31 : xbsIndex_r4/Convert  gui_display_data_type=Fixed-point  arith_type=Unsigned  n_bits=5  bin_pt=0  float_type=Single  exp_bits=8  fraction_bits=24  quantization=Truncate  overflow=Saturate  en=off  latency=0  dbl_ovrd=off  pipeline=off  block_type=convert
  depth 7 : xbsIndex_r4/Convert  gui_display_data_type=Fixed-point  arith_type=Unsigned  n_bits=3  bin_pt=0  float_type=Single  exp_bits=8  fraction_bits=24  quantization=Truncate  overflow=Saturate  en=off  latency=0  dbl_ovrd=off  pipeline=off  block_type=convert
  rising edge : Subsystem
  SPIWrite_Start : Outport
  SPIWrite_Data : Outport  Port=2
  GainSetMaster_Done : Outport  Port=3
  Current_Gain_Setting : Outport  Port=4
  SoftSPIBusy : Outport  Port=5
  tag scope: cs_currentgainsetting=global, cs_spi_data=global, cs_spi_start=global
  wires:
  To Register/1 -> depth 31/1, Ufix8_to_fix9_1/1
  To Register1/1 -> depth 26/1, Ufix8_to_fix9_3/1
  To Register2/1 -> depth 7/1, Ufix8_to_fix9_2/1
  Gain_Setting_ROM/1 -> K_RxVGA2_Bit[8..16]/1, J_RxVGA1_Bit[0..7]/1, L_LNA_Bit[17..24]/1  "req_gain_settings"
  GainSetMaster_TargetGain/1 -> Gain_Setting_ROM/1
  Delay/1 -> To Register/2, To Register1/2, To Register2/2, Delay1/1
  depth 7/1 -> L_RxLNA_Code_ROM/1
  depth 26/1 -> J_RxVGA1_Code_ROM/1
  depth 31/1 -> K_RxVGA2_Code_ROM/1
  Delay1/1 -> Delay2/1
  Delay2/1 -> SPI_Controller1/1(Start)
  K_RxVGA2_Code_ROM/1 -> SPI_Controller1/2(RxVGA2_Code)
  J_RxVGA1_Code_ROM/1 -> SPI_Controller1/3(RxVGA1_Code)
  L_RxLNA_Code_ROM/1 -> SPI_Controller1/4(RxLNA_Code)
  SPI_Controller1/1(SPIWrite_Start) -> [cs_spi_start], [debug_spiWriteStart], SPIWrite_Start/1
  SPI_Controller1/2(SPWrite_Frame) -> [cs_spi_data], [debug_spiWriteData], SPIWrite_Data/1
  SPI_Controller1/3(Done) -> GainSetMaster_Done/1, SR-Latch/2(R)
  rising edge/1(Q) -> [debug_gainSetStart], Delay/1
  Ufix8_to_fix9_1/1 -> AddSub2/1
  Ufix8_to_fix9_3/1 -> AddSub2/2
  AddSub2/1 -> AddSub3/1
  Ufix8_to_fix9_2/1 -> AddSub3/2
  AddSub3/1 -> [cs_currentgainsetting], Current_Gain_Setting/1  "Current Gain"
  Mux3/1 -> To Register/1
  Mux4/1 -> To Register1/1
  K_RxVGA2_Bit[8..16]/1 -> Mux3/3
  J_RxVGA1_Bit[0..7]/1 -> Mux4/3
  Mux5/1 -> To Register2/1
  L_LNA_Bit[17..24]/1 -> Mux5/3
  AGC_Enable/1 -> Mux4/1, Mux5/1, Mux3/1, SPI_Controller1/5(AGC_Enable)  "AGC_Enable"
  [regAGC_ManualRxVGA2_Gain] -> Mux3/2
  [regAGC_ManualRxVGA1_Gain] -> Mux4/2
  [regAGC_ManualRxLNA_Gain] -> Mux5/2
  Logical3/1 -> rising edge/1(A)
  [regAGC_softGainWrite] -> Logical3/1
  GainSetMaster_Go/1 -> [SPIGO], Logical3/2
  DynDef Trigger/1 -> Delay3/1
  Delay3/1 -> Delay4/1
  Delay4/1 -> Delay5/1
  Delay5/1 -> SPI_Controller1/6(DynDef Trigger)
  SR-Latch/1(Q) -> [debug_softSPIBusy], SoftSPIBusy/1
  [SPIGO] -> SR-Latch/1(S)
